simulink model "SOE_H2_DRI_plant"  (R2023b)
settings: Solver=ode15s  StartTime=0.0  StopTime=3600*24*8759
values from neighbouring files (symbols this model uses):
  a_b = 6*(1-eps_bed)/(r_p*2)    (= 200)    [H2_DRI_plant_loader.m]
  A_furnace = pi*r_furnace^2    (= 23.7582944428)    [H2_DRI_plant_loader.m]
  A_furnace_pel = A_furnace*(1-eps_bed)    (= 11.8791472214)    [H2_DRI_plant_loader.m]
  A_wall = (2*pi*r_furnace*dz)    (= 1.1674837564)    [H2_DRI_plant_loader.m]
  c_CH4init = interp1([1:1:length(c_CH4init)],c_CH4init, linspace(1,length(c_CH4init),n_furnace))    [H2_DRI_plant_loader.m]    (also in inital_conditions.m = out.CH4_conc.data(end,:); initcond_H2.mat = [9.94099064213e-45 -4.26076213273e-25 -4.27813906239e-25 -4.; initcond_H2_PEM.mat = [4.30667282687e-45 4.29087427587e-45 3.8700760922e-45 3.7994)
  c_Cinit = interp1([1:1:length(c_Cinit)],c_Cinit, linspace(1,length(c_Cinit),n_furnace))    [H2_DRI_plant_loader.m]    (also in inital_conditions.m = out.C_conc.data(end,:); initcond_H2.mat = [1.45956980986e-305 6.99081092012e-307 8.03725154841e-309 -3; initcond_H2_PEM.mat = [1.92191536232e-321 1.91203404941e-321 1.97132192691e-321 1.)
  c_CO2init = interp1([1:1:length(c_CO2init)],c_CO2init, linspace(1,length(c_CO2init),n_furnace))    [H2_DRI_plant_loader.m]    (also in inital_conditions.m = out.CO2_conc.data(end,:); initcond_H2.mat = [1.40671287015e-53 9.99429922421e-25 1.00349747704e-24 1.007; initcond_H2_PEM.mat = [4.30579616214e-45 4.28998535938e-45 3.86916279543e-45 3.798)
  c_COinit = interp1([1:1:length(c_COinit)],c_COinit, linspace(1,length(c_COinit),n_furnace))    [H2_DRI_plant_loader.m]    (also in inital_conditions.m = out.CO_conc.data(end,:); initcond_H2.mat = [8.62168160047e-54 2.62488347241e-25 2.63562031881e-25 2.646; initcond_H2_PEM.mat = [-1.41770643933e-43 -1.41248114323e-43 -1.27321677334e-43 -1)
  c_Fe2O3init = interp1([1:1:length(c_Fe2O3init)],c_Fe2O3init, linspace(1,length(c_Fe2O3init),n_furnace))    [H2_DRI_plant_loader.m]    (also in inital_conditions.m = out.Fe2O3_conc.data(end,:); initcond_H2.mat = [-0.0576294325141 -0.0562977053664 -0.0549879883395 -0.05369; initcond_H2_PEM.mat = [-0.0421766495112 -0.0410731169681 -0.0399918101679 -0.03893)
  c_Fe3O4init = interp1([1:1:length(c_Fe3O4init)],c_Fe3O4init, linspace(1,length(c_Fe3O4init),n_furnace))    [H2_DRI_plant_loader.m]    (also in inital_conditions.m = out.Fe3O4_conc.data(end,:); initcond_H2.mat = [0.0460784397936 0.0452182842983 0.0443654100081 0.043519007; initcond_H2_PEM.mat = [0.0345314201173 0.0338401633931 0.0331554273597 0.032476466)
  c_Feinit = interp1([1:1:length(c_Feinit)],c_Feinit, linspace(1,length(c_Feinit),n_furnace))    [H2_DRI_plant_loader.m]    (also in inital_conditions.m = out.Fe_conc.data(end,:); initcond_H2.mat = [2291.15615825 2257.57098555 2219.35021937 2176.85237423 213; initcond_H2_PEM.mat = [2291.15370188 2257.40533074 2219.07663621 2176.56351656 213)
  c_FeOinit = interp1([1:1:length(c_FeOinit)],c_FeOinit, linspace(1,length(c_FeOinit),n_furnace))    [H2_DRI_plant_loader.m]    (also in inital_conditions.m = out.FeO_conc.data(end,:); initcond_H2.mat = [120.587032003 163.793602795 212.96382844 267.636483226 327.; initcond_H2_PEM.mat = [120.587036941 164.003608886 213.312732219 268.005087273 327)
  c_H2init = interp1([1:1:length(c_H2init)],c_H2init, linspace(1,length(c_H2init),n_furnace))    [H2_DRI_plant_loader.m]    (also in inital_conditions.m = out.H2_conc.data(end,:); initcond_H2.mat = [22.889073739 22.8842667021 22.8746324515 22.8599710419 22.8; initcond_H2_PEM.mat = [17.1469199078 17.1645959742 17.1787956185 17.1891948084 17.)
  c_H2Oinit = interp1([1:1:length(c_H2Oinit)],c_H2Oinit, linspace(1,length(c_H2Oinit),n_furnace))    [H2_DRI_plant_loader.m]    (also in inital_conditions.m = out.H2O_conc.data(end,:); initcond_H2.mat = [2.19324064628 2.2939246227 2.40633645516 2.52967076126 2.66; initcond_H2_PEM.mat = [0.652099757837 0.728496202531 0.813916572535 0.907739128718)
  c_N2init = interp1([1:1:length(c_N2init)],c_N2init, linspace(1,length(c_N2init),n_furnace))    [H2_DRI_plant_loader.m]    (also in inital_conditions.m = out.N2_conc.data(end,:); initcond_H2.mat = [0.439764167248 0.441445162144 0.443247144888 0.445152489232; initcond_H2_PEM.mat = [0.271051060899 0.272483637209 0.274000693264 0.275587826454)
  cCarbon = 180/1000    (= 0.18)    [H2_DRI_plant_loader.m]
  CCcomp = 6151202*Pcomp^0.71    (= 33253176.5742)    [H2_DRI_plant_loader.m]
  CCeaf = 160*ls_prod_kg*8760/1000    (= 151726003.2)    [H2_DRI_plant_loader.m]
  CCelect = CC_elect*MWelect*1000    (= 480904000)    [H2_DRI_plant_loader.m]
  CCfur = 228860*Qfurnace^0.7848    (= 4163876.6695)    [H2_DRI_plant_loader.m]
  CCpsa = 30622*m_O2^0.6357    (= 6771939.09833)    [H2_DRI_plant_loader.m]
  CCsf = 250*ls_prod_kg*8760/1000    (= 237071880)    [H2_DRI_plant_loader.m]
  cLime = 100/1000    (= 0.1)    [H2_DRI_plant_loader.m]
  cNG = 7    [H2_DRI_plant_loader.m]
  CO2_diff_prop = [MM_CO2, 26.9]    [H2_DRI_plant_loader.m]
  CO_diff_prop = [MM_CO, 18.9]    [H2_DRI_plant_loader.m]
  D_metal = 0.5*I_metal    (= -0.0319284802043)    [H2_DRI_plant_loader.m]
  DRIsteel_conv = 1.075    [H2_DRI_plant_loader.m]
  dz = (h_furnace/(n_furnace-1))    (= 0.0675675675676)    [H2_DRI_plant_loader.m]
  EAF_elec_req = 375    [H2_DRI_plant_loader.m]
  eps_bed = 0.5    [H2_DRI_plant_loader.m]
  eta_comb = 0.8    [H2_DRI_plant_loader.m]
  eta_isen = 0.75    [H2_DRI_plant_loader.m]
  eta_motor = 0.95    [H2_DRI_plant_loader.m]
  H2_diff_prop = [MM_H2, 2.31*2]    [H2_DRI_plant_loader.m]
  H2O_diff_prop = [MM_H2O, 13.1]    [H2_DRI_plant_loader.m]
  H2only = true    [H2_DRI_plant_loader.m]
  hot_standby_eff = 0.009    [H2_DRI_plant_loader.m]
  I_metal = P_metal/tau_metal    (= -0.0638569604087)    [H2_DRI_plant_loader.m]
  Kd = 0.00728    [H2_DRI_plant_loader.m]
  Kmetal = -0.0435    [H2_DRI_plant_loader.m]
  labor_cost = 19*DRI_prod_kg/3600/1000 + 53*ls_prod_kg/3600/1000    (= 2.20779)    [H2_DRI_plant_loader.m]
  m_O2rate = 45.072    [H2_DRI_plant_loader.m]
  MM_C = 12.011/1000    (= 0.012011)    [H2_DRI_plant_loader.m]
  MM_CH4 = 16.04    [H2_DRI_plant_loader.m]
  MM_CO = 28.01    [H2_DRI_plant_loader.m]
  MM_CO2 = 44.01    [H2_DRI_plant_loader.m]
  MM_Fe = 55.845/1000    (= 0.055845)    [H2_DRI_plant_loader.m]    (also in iron_props.m)
  MM_Fe2O3 = 159.69/1000    (= 0.15969)    [H2_DRI_plant_loader.m]    (also in iron_props.m)
  MM_Fe3O4 = 231.53/1000    (= 0.23153)    [H2_DRI_plant_loader.m]    (also in iron_props.m = 0.25153)
  MM_FeO = 71.844/1000    (= 0.071844)    [H2_DRI_plant_loader.m]    (also in iron_props.m)
  MM_H2 = 2.016    [H2_DRI_plant_loader.m]
  MM_H2O = 18.015    [H2_DRI_plant_loader.m]
  MM_N2 = 28.013    [H2_DRI_plant_loader.m]
  MWelect = 240.452    [H2_DRI_plant_loader.m]
  MWhNGeaf = 0.08792    [H2_DRI_plant_loader.m]
  n_furnace = 75    [H2_DRI_plant_loader.m]
  ndot_H2O_feed = linspace(35, 155, n_loops)    [RTO_model_datapoints.m]
  ndot_path = ndot_path(:,3)    [H2_DRI_plant_loader.m]
  ndotin = 2706    [H2_DRI_plant_loader.m]
  nr1init = interp1([1:1:length(nr1init)],nr1init, linspace(1,length(nr1init),n_furnace))    [H2_DRI_plant_loader.m]    (also in inital_conditions.m = out.nr1.data(end,:); initcond_H2.mat = [17138.9259823 17138.9192887 17138.9127057 17138.9062259 171; initcond_H2_PEM.mat = [17138.8483125 17138.8427658 17138.8373309 17138.8319998 171)
  nr2init = interp1([1:1:length(nr2init)],nr2init, linspace(1,length(nr2init),n_furnace))    [H2_DRI_plant_loader.m]    (also in inital_conditions.m = out.nr2.data(end,:); initcond_H2.mat = [11425.7909148 11425.7894343 11425.7880023 11425.7866166 114; initcond_H2_PEM.mat = [11425.7791649 11425.7778635 11425.776614 11425.7754137 1142)
  nr3init = interp1([1:1:length(nr3init)],nr3init, linspace(1,length(nr3init),n_furnace))    [H2_DRI_plant_loader.m]    (also in inital_conditions.m = out.nr3.data(end,:); initcond_H2.mat = [32930.1678524 32447.4572478 31898.1205118 31287.3104766 306; initcond_H2_PEM.mat = [32930.1325476 32445.0763361 31894.188375 31283.1588034 3061)
  oxy_eff_tonne = 0.803    [H2_DRI_plant_loader.m]
  P_g_sp = 101325*2.5    (= 253312.5)    [H2_DRI_plant_loader.m]
  P_metal = tau_metal/(Kmetal*tau_metal_desired)    (= -735.632183908)    [H2_DRI_plant_loader.m]
  pandcdata = csvread('caiso_lmp_carbon_clean.csv', 1, 1)    [H2_DRI_plant_loader.m]
  R = 8.314    [Bou.m]    (also in H2_DRI_plant_loader.m; MD.m; SMR.m; USCM_CO.m)
  r_furnace = 2.75    [H2_DRI_plant_loader.m]
  r_p = 15e-3/2    (= 0.0075)    [H2_DRI_plant_loader.m]
  rho_p = 3528    [H2_DRI_plant_loader.m]
  SOEeff = 37.5    [H2_DRI_plant_loader.m]
  stack_replace = 3.25    [H2_DRI_plant_loader.m]
  T_gin = 950 + 273    (= 1223)    [H2_DRI_plant_loader.m]
  T_ginit = interp1([1:1:length(T_ginit)],T_ginit, linspace(1,length(T_ginit),n_furnace))    [H2_DRI_plant_loader.m]    (also in inital_conditions.m = out.T_g.data(end,2:end); initcond_H2.mat = [1193.47241077 1188.60147936 1183.4413554 1178.04610025 1172; initcond_H2_PEM.mat = [1213.62674902 1206.86882145 1199.80656651 1192.51337179 118)
  T_sin = 10 + 273    (= 283)    [H2_DRI_plant_loader.m]
  T_sinit = interp1([1:1:length(T_sinit)],T_sinit, linspace(1,length(T_sinit),n_furnace))    [H2_DRI_plant_loader.m]    (also in inital_conditions.m = out.T_s.data(end,1:end-1); initcond_H2.mat = [1188.32225462 1183.11411515 1177.66723955 1172.0331792 1166; initcond_H2_PEM.mat = [1207.76768382 1200.67884676 1193.34151616 1185.82650883 117)
  tau = 1    [H2_DRI_plant_loader.m]
  tau_d = 3600    [H2_DRI_plant_loader.m]
  tau_metal = 3.2*3600    (= 11520)    [H2_DRI_plant_loader.m]
  taxes = tax_rate*TIC/8760/3600    [H2_DRI_plant_loader.m]
  V_g = (4/3)*pi*r_p^3*n_pellets_dz*(eps_bed/(1-eps_bed))    (= 0.802645082526)    [H2_DRI_plant_loader.m]
  V_p = 4/3*pi*r_p^3    (= 1.76714586764e-06)    [H2_DRI_plant_loader.m]
  V_s = (4/3)*pi*r_p^3*n_pellets_dz    (= 0.802645082526)    [H2_DRI_plant_loader.m]
  w_Cin = 0    [H2_DRI_plant_loader.m]
  w_Fe2O3in = 0.9665    [H2_DRI_plant_loader.m]
  w_Fe3O4in = 0    [H2_DRI_plant_loader.m]
  w_Fein = 0    [H2_DRI_plant_loader.m]
  w_FeOin = 0    [H2_DRI_plant_loader.m]
  w_Ganin = 0.0335    [H2_DRI_plant_loader.m]
  x_H2in = 0.90    (= 0.9)    [H2_DRI_plant_loader.m]
  x_H2Oin = 0.085    [H2_DRI_plant_loader.m]
  x_N2in = 0.015    [H2_DRI_plant_loader.m]
undefined symbols (not defined in the file or in its folder): CCbop
libraries: slpidlib x2
(part 3 of 3)

== matlab function SOE_H2_DRI_plant/DRI Shaft Furnace/solid_conc ==
  data: rho_Fe2O3in output; w_Fe2O3 input; w_Fe3O4 input; w_FeO input; w_Fe input; w_C input; w_Gan input; m_solid input; rho_Fe3O4in output; rho_FeOin output; A_furnace parameter; rho_Fein output; rho_Cin output; rho_Ganin output; u_sin output; rho_p parameter; eps_bed parameter; pellet_flow output; r_p parameter
function [rho_Fe2O3in, rho_Fe3O4in, rho_FeOin, rho_Fein, rho_Cin, rho_Ganin, u_sin, pellet_flow] = solid_conc(w_Fe2O3, w_Fe3O4, w_FeO, w_Fe, w_C, w_Gan, m_solid, A_furnace,rho_p, eps_bed, r_p)

%toal mass concentration using ped porosity and density of pellet
rho_bedin = rho_p; %kg/^3 of SOLID

%mass concentrations of each iron species in
rho_Fe2O3in = rho_bedin * w_Fe2O3; %kg/m^3 of pellet
rho_Fe3O4in = rho_bedin * w_Fe3O4; %kg/m^3 of pellet
rho_FeOin = rho_bedin * w_FeO; %kg/m^3 of pellet
rho_Fein = rho_bedin * w_Fe; %kg/m^3 of pellet
rho_Cin = rho_bedin * w_C; %kg/m^3 of pellet
rho_Ganin = rho_bedin * w_Gan; %kg/m^3 of pellet


%vol_flow = m_solid/(rho_bedin*(1-eps_bed)); %m^3 total/s

u_sup = m_solid/(rho_p*A_furnace);%*(1-eps_bed));

            
u_sin = u_sup/(1-eps_bed);

%interstitial velocity of mass flow, m/s
%u_sin = m_solid/rho_bedin/(A_furnace*(1-eps_bed));


%check this!
pellet_flow = (3*m_solid)/(4*pi*r_p^3*rho_bedin); %pellets/s

== matlab function SOE_H2_DRI_plant/Electrolyzer/SOE ==
  data: T_gin input; ndot_in input; x_H2in input; x_H2Oin input; x_N2in input; T_gout output; SOEeff parameter; ndot_out output; x_H2out output; x_H2Oout output; x_N2out output; ndot_O2_prod output; MM_H2 parameter; MM_H2O parameter; MM_N2 parameter; MWelect output
function [T_gout, ndot_out, x_H2out, x_H2Oout, x_N2out, ndot_O2_prod, MWelect] = SOE(T_gin, ndot_in, x_H2in, x_H2Oin, x_N2in, SOEeff, MM_H2, MM_H2O, MM_N2)

% mdot_H2_prod = MWelect/(SOEeff*3.6); % kg/s H2 prod
% ndot_H2_prod = mdot_H2_prod/(MM_H2/1000); %mol/s H2 prod
% 
% ndot_O2_prod = 0.5*ndot_H2_prod; %mol/s H2 prod
% ndot_H2O_react = ndot_H2_prod;
% 
% 
% moles_H2 = ndot_in*x_H2in + ndot_H2_prod;
% moles_H2O = ndot_in*x_H2Oin - ndot_H2O_react;
% moles_N2 = ndot_in*x_N2in ;

ndot_out = ndot_in;
x_H2out = 0.89;

ndot_H2_prod = ndot_out*x_H2out - ndot_in*x_H2in;

ndot_O2_prod = 0.5*ndot_H2_prod; %mol/s H2 prod
ndot_H2O_react = ndot_H2_prod;

moles_H2O = ndot_in*x_H2Oin - ndot_H2O_react;
moles_N2 = ndot_in*x_N2in ;


x_H2Oout = moles_H2O/ndot_out;
x_N2out = moles_N2/ndot_out;

T_gout = T_gin + 15;

% mdot_H2_prod = MWelect/(SOEeff*3.6); % kg/s H2 prod
mdot_H2_prod = ndot_H2_prod*MM_H2/1000; %kg/s H2 produced

MWelect = mdot_H2_prod*(SOEeff*3.6); %MW required to react this much

== matlab function SOE_H2_DRI_plant/Splitter/splitter ==
  data: ndotin input; purgefraction input; ndot_comp output; ndot_purge output
function [ndot_comp, ndot_purge] = splitter(ndotin, purgefraction)

ndot_purge = purgefraction*ndotin;
ndot_comp = ndotin*(1-purgefraction);

== matlab function SOE_H2_DRI_plant/Recycle Compressor/compressor ==
  data: P_g_sp input; P_gin input; P_gout output; T_gin input; T_gout output; ndot input; x_H2 input; x_H2O input; x_N2 input; MWcomp output; eta_isen parameter; R parameter; eta_motor parameter; MM_H2O parameter; MM_H2 parameter; MM_N2 parameter
function [P_gout, T_gout, MWcomp] = compressor(P_g_sp, P_gin, T_gin, ndot, x_H2, x_H2O, x_N2, eta_isen, R, eta_motor, MM_H2O, MM_H2, MM_N2)

npoly = 1.4;
P_gout = P_g_sp;


mdot = ndot*(x_H2*MM_H2  + x_H2O*MM_H2O + x_N2*MM_N2)/1000; %kg/s
R_g = R/(x_H2*MM_H2  + x_H2O*MM_H2O + x_N2*MM_N2)*1000; %J/kg-K


%%


W = mdot*(npoly/(npoly-1))*R_g*T_gin*((P_gout/P_gin)^((npoly-1)/npoly) - 1);
MWcomp = W/(eta_isen*eta_motor)/1e6;


T_gout = T_gin*(P_gout/P_gin)^((npoly-1)/npoly);

== matlab function SOE_H2_DRI_plant/Direct Injection Steam Generator/MATLAB Function ==
  data: P_f input; P_gout output; T_gout output; T_f input; ndot_f input; ndotout output; x_H2out output; x_H2Oout output; x_N2out output; P_r input; T_r input; ndot_r input; x_H2_r input; x_H2O_r input; x_N2_r input; MM_H2 parameter; MM_N2 parameter; MM_H2O parameter
function [P_gout, T_gout, ndotout, x_H2out, x_H2Oout, x_N2out] ...
    = steam_gen(P_f, T_f, ndot_f,...
               P_r, T_r, ndot_r, x_H2_r, x_H2O_r, x_N2_r, MM_H2, MM_N2, MM_H2O)

ndotout = ndot_f + ndot_r;

%T_gout = T_r; %need to update using specific heats

P_gout = (ndot_f*P_f + ndot_r*P_r)/(ndotout);

moles_H2 = ndot_r*x_H2_r;
moles_H2O = ndot_r*x_H2O_r + ndot_f;
moles_N2 = ndot_r*x_N2_r ;

x_H2out = moles_H2/ndotout;
x_H2Oout = moles_H2O/ndotout;
x_N2out = moles_N2/ndotout;

%% Recycle Stream

mdot_r = ndot_r*(x_H2_r*MM_H2 + x_N2_r*MM_N2 + x_H2O_r*MM_H2O)/1000; %kg/s

% Weight fractions of each gas species
w_tot_r = (x_H2_r*MM_H2 + x_H2O_r*MM_H2O + x_N2_r*MM_N2);

w_H2_r = x_H2_r*MM_H2/w_tot_r;
w_H2O_r = x_H2O_r*MM_H2O /w_tot_r;
w_N2_r = x_N2_r*MM_N2/w_tot_r;

w_fracs_r = [w_H2_r, w_H2O_r, w_N2_r]; % Create a vector of weight fractions for the prop_mix function

% Get properties from CoolProp interpolation based on temp of gas in
[H_H2, mu_H2, k_H2, C_H2] = hydrogen(T_r);
[H_H2O, mu_H2O, k_H2O, C_H2O] = water(T_r);
[H_N2, mu_N2, k_N2, C_N2] = nitrogen(T_r);


% Create vectors of properties for prop_mix function
Hs = [H_H2, H_H2O, H_N2];
mus = [mu_H2, mu_H2O, mu_N2];
ks = [k_H2, k_H2O, k_N2];
Cps = [C_H2, C_H2O, C_N2];

% get vicosicty and specific heat of gas mixture in
[H_r, ~, ~,  ~] = prop_mix(Hs, mus, ks, Cps, w_fracs_r);

h_r = H_r*mdot_r; % W, enthalpy of recycle stream

%% Water Stream

[H_f, ~, ~,~] = water(T_f);
mdot_f = ndot_f*MM_H2O/1000;
h_f = H_f*mdot_f; % W, enthalpy of feed stream

%% Mixed Enthalpy

H_mix_target = (h_r + h_f)/(mdot_r + mdot_f); %J/kg

%% Out Enthalpy

mdotout = ndotout*(x_H2out*MM_H2 + x_N2out*MM_N2 + x_H2Oout*MM_H2O)/1000; %kg/s

% Weight fractions of each gas species
w_totout = (x_H2out*MM_H2 + x_H2Oout*MM_H2O + x_N2out*MM_N2);

w_H2out = x_H2out*MM_H2/w_totout;
w_H2Oout = x_H2Oout*MM_H2O /w_totout;
w_N2out = x_N2out*MM_N2/w_totout;

w_fracsout = [w_H2out, w_H2Oout, w_N2out]; % Create a vector of weight fractions for the prop_mix function

T_low = 100+273;
T_high = 1000;
tol = 1; 
max_iter = 10000;

T_gout = bisection_method(T_low, T_high, tol, max_iter, w_fracsout, H_mix_target);

== matlab function SOE_H2_DRI_plant/DRI Shaft Furnace/Mixer/MATLAB Function ==
  data: P_gin_f input; P_gout output; T_gout output; T_gin_f input; ndotin_f input; x_H2in_f input; x_H2Oin_f input; x_N2in_f input; x_COin_f input; x_CO2in_f input; x_CH4in_f input; ndotout output; x_H2out output; x_H2Oout output; x_N2out output; x_COout output; x_CO2out output; x_CH4out output; ndotin_N2extra input
function [P_gout, T_gout, ndotout, x_H2out, x_H2Oout, x_N2out, x_COout, x_CO2out, x_CH4out] ...
    = mixer(P_gin_f, T_gin_f, ndotin_f, x_H2in_f, x_H2Oin_f, x_N2in_f, x_COin_f, x_CO2in_f, x_CH4in_f, ndotin_N2extra)

ndotout = ndotin_f + ndotin_N2extra;

T_gout = T_gin_f; %need to update using specific heats

P_gout = P_gin_f;

moles_H2 = ndotin_f*x_H2in_f;
moles_H2O = ndotin_f*x_H2Oin_f;
moles_N2 = ndotin_f*x_N2in_f + ndotin_N2extra;
moles_CO = ndotin_f*x_COin_f;
moles_CO2 = ndotin_f*x_CO2in_f;
moles_CH4 = ndotin_f*x_CH4in_f;

x_H2out = moles_H2/ndotout;
x_H2Oout = moles_H2O/ndotout;
x_N2out = moles_N2/ndotout;
x_COout = moles_CO/ndotout;
x_CO2out = moles_CO2/ndotout;
x_CH4out = moles_CH4/ndotout;

== matlab function SOE_H2_DRI_plant/Combustion Furnace/MATLAB Function ==
  data: ndot input; x_H2 input; x_H2O input; x_N2 input; T_g input; Q_heat output; T_gsp input; MM_H2O parameter; MM_H2 parameter; MM_N2 parameter; mdot output; Cp_g output
function [Q_heat, mdot, Cp_g] = furnace(ndot, x_H2, x_H2O, x_N2, T_g, T_gsp, MM_H2O, MM_H2, MM_N2)

T_g_mid = (T_g + T_gsp)/2;

mdot = ndot*(x_H2*MM_H2 + x_H2O*MM_H2O+ x_N2*MM_N2)/1000; %kg/s

% Weight fractions of each gas species
w_totin = (x_H2*MM_H2 + x_H2O*MM_H2O + x_N2*MM_N2);

w_H2in = x_H2*MM_H2/w_totin;
w_H2Oin = x_H2O*MM_H2O /w_totin;
w_N2in = x_N2*MM_N2/w_totin;


w_fracs = [w_H2in, w_H2Oin, w_N2in]; % Create a vector of weight fractions for the prop_mix function

% Get properties from CoolProp interpolation based on temp of gas in
[rho_H2, mu_H2, k_H2, C_H2] = hydrogen(T_g_mid);
[rho_H2O, mu_H2O, k_H2O, C_H2O] = water(T_g_mid);
[rho_N2, mu_N2, k_N2, C_N2] = nitrogen(T_g_mid);


% Create vectors of properties for prop_mix function
rhos = [rho_H2, rho_H2O, rho_N2];
mus = [mu_H2, mu_H2O, mu_N2];
ks = [k_H2, k_H2O, k_N2];
Cps = [C_H2, C_H2O, C_N2];

% get vicosicty and specific heat of gas mixture in
[~, ~, ~,  Cp_g] = prop_mix(rhos, mus, ks, Cps, w_fracs);

Q_heat = mdot*Cp_g*(T_gsp - T_g)/1e6;

== matlab function SOE_H2_DRI_plant/Combustion Furnace/MATLAB Function1 ==
  data: ndot_p input; Q_purge output; x_H2_p input; x_H2O_p input; x_N2_p input; MM_H2O parameter; MM_H2 parameter; MM_N2 parameter; mdot_p output
function [Q_purge, mdot_p] = purge_comb(ndot_p, x_H2_p, x_H2O_p, x_N2_p, MM_H2O, MM_H2, MM_N2)

Q_purge =  ndot_p*x_H2_p*238440/1e6;

mdot_p = ndot_p*(x_H2_p*MM_H2 + x_H2O_p*MM_H2O+ x_N2_p*MM_N2)/1000; %kg/s

== matlab function SOE_H2_DRI_plant/MATLAB Function ==
  data: LCOE input; elec_CO2rate input; cIO input; pLS input; MWelect input; MWeaf input; MWcomp input; MWpsa input; MWcooltow input; LCOS output; MWng input; MWng_eaf input; m_IO input; m_steel input; carbon_consume input; lime_consume input; CCeaf parameter; CCelect parameter; CCsf parameter; LCOS_bd output; SCE output; SCE_bd output; CCbop parameter; taxes parameter; labor_cost parameter; cNG parameter; cCarbon parameter; cLime parameter; stack_replace parameter; profit output; emissions_profit output; CCfur parameter; CCpsa parameter; CCcomp parameter; cost output; emissions output; MWe output; CCcooltow input
function [LCOS, LCOS_bd, SCE, SCE_bd, profit, emissions_profit, cost, emissions, MWe] = LCOS( LCOE, elec_CO2rate, cIO, pLS, MWelect, MWeaf, MWcomp, MWpsa, MWcooltow, MWng, MWng_eaf,m_IO, m_steel, carbon_consume, lime_consume, ...
    CCeaf, CCelect, CCsf, CCbop, taxes, labor_cost, cNG, cCarbon, cLime, stack_replace, CCfur, CCpsa, CCcomp, CCcooltow)


% m_steel = tonne liquid steel per second

%==========================Variable O&M==============================


io_cost = m_IO*cIO/1000; % $/s, cost of iron ore
MWe = (MWelect+MWeaf+MWcomp+MWpsa+MWcooltow);
elec_cost = (MWelect+MWeaf+MWcomp+MWpsa+MWcooltow)*LCOE/3600; % $/s, cost of electricity
gas_cost = (MWng + MWng_eaf) *3.412*cNG/3600; % $/s, cost of ng

carbon_cost = carbon_consume*cCarbon; %$, cost of carbon
lime_cost = lime_consume*cLime; % cost of lime

stack_cost = MWelect*0.975*stack_replace/3600; % $/s %0.975 is rectifier efficiency - cost to replace stacks


%% LCOS
%CRF = 0.136;
CRF = 0.1019;
%CRF = 0.0776;


CCann = (CCeaf + CCelect + CCsf + CCfur + CCcomp + CCpsa + CCcooltow + CCbop)*CRF;
CC_cost = CCann/(8760*3600); % $/s for plant capital costs

%tax_cost = tax_rate*(CC_cost/CRF +labor_cost); % $/s 

LCOS = (io_cost + elec_cost + gas_cost + CC_cost + taxes + labor_cost + carbon_cost + lime_cost + stack_cost)/m_steel;

cost = (io_cost + elec_cost + gas_cost + CC_cost + taxes + labor_cost + carbon_cost + lime_cost + stack_cost);
revenue = m_steel*pLS;

profit  = revenue - cost;

LCOS_bd = [CCelect*CRF/(8760*3600) CCsf*CRF/(8760*3600) CCeaf*CRF/(8760*3600) ...
    CCfur*CRF/(8760*3600) CCcomp*CRF/(8760*3600) CCpsa*CRF/(8760*3600) CCcooltow*CRF/(8760*3600) CCbop*CRF/(8760*3600)...
    elec_cost  gas_cost  io_cost  carbon_cost + lime_cost + stack_cost labor_cost taxes ]/m_steel;

% ==========================CO2 Emissions==============================
% 
ng_CO2rate = 198; %kg CO2/MWh nat gas -from my 1st paper
ng_CO2rate_us = 47; %kg CO2e nat upstream - from Incentives for Clean Hydrogen Production in the Inflation Reduction Act

lime_CO2rate = 0.05; %kg CO2/kg lime consumed
carbon_CO2rate = 0.98; %kg CO2/kg carbon consumed
io_CO2rate = 0.02; %kg CO2/kg iron ore
pell_CO2rate = 0.16; %kg CO2/kg iron ore
og_CO2rate = 0.101; %kg CO2/kg ls
% 
elec_CO2 = (MWelect+MWeaf+MWcomp+MWpsa+MWcooltow)*elec_CO2rate/3600; %kg CO2/s from electricity
ng_CO2 = (MWng + MWng_eaf)*ng_CO2rate/3600; % kg CO2/s from natural gas combustion
 
EAFog_CO2 = og_CO2rate*m_steel*1000;  %kg CO2/s from combustion of EAF off gas
ng_CO2us = (MWng + MWng_eaf)*ng_CO2rate_us/3600; %kg CO2/s from upstream natural gas use


lime_CO2 = lime_CO2rate*lime_consume; %kg CO2/s from lime production
carbon_CO2 = carbon_CO2rate*carbon_consume; %kg CO2/s from coal/coke production
io_CO2 = io_CO2rate*m_IO; %kg CO2/yr from iron ore mining
pell_CO2 = pell_CO2rate*m_IO;  %kg CO2/yr from iron ore pelletizing
mineralCO2 = lime_CO2 + carbon_CO2 + io_CO2; %kg CO2/yr from mineral production/mining excluding pelletizing

SCE = (elec_CO2 + ng_CO2 + EAFog_CO2 + ng_CO2us + pell_CO2 + mineralCO2)/m_steel/1000; % t CO2e/ t ls
SCE_bd = [ng_CO2  EAFog_CO2  elec_CO2  ng_CO2us   pell_CO2  mineralCO2]/m_steel/1000; % t CO2e/ t ls

emissions = (elec_CO2 + ng_CO2 + EAFog_CO2 + ng_CO2us + pell_CO2 + mineralCO2); %kg/s
emissions_goal = m_steel*1.32*1000; %kg/s

emissions_profit = emissions_goal - emissions;

== matlab function SOE_H2_DRI_plant/Subsystem/EAF ==
  data: m_steel output; m_DRI input; MWeaf output; DRIsteel_conv parameter; EAF_elec_req parameter; MWpsa output; MWng_eaf output; m_O2rate parameter; oxy_eff_tonne parameter; carbon_consume output; lime_consume output; MWhNGeaf parameter
function [m_steel, MWeaf, MWpsa, MWng_eaf, carbon_consume, lime_consume] = eaf(m_DRI, DRIsteel_conv, EAF_elec_req, m_O2rate, oxy_eff_tonne, MWhNGeaf)

m_steel = m_DRI/DRIsteel_conv/1000; %tonne/s steel
m_O2 = m_O2rate*m_steel; %kg/s O2 req
m_O2tonne = m_O2*3.6; % tonne/hr O2 required


MWpsa =  m_O2tonne*oxy_eff_tonne; 

MWeaf = EAF_elec_req*m_steel*3.6; % MWe for EAF

MWng_eaf = MWhNGeaf*m_steel*3600;

%lime and carbon consumption
carbon_consume = 27*m_steel; % kg/s, (kg/tonne ls * tonne_ls)
lime_consume = 50*m_steel; % kg/s, (kg/tonne ls * tonne_ls)

== matlab function SOE_H2_DRI_plant/Direct Injection Steam Generator/MATLAB Function1 ==
  data: time input; ndot_H2O output; ndot_path parameter; t parameter
function ndot_H2O  = interpolator(time, ndot_path, t)

%t = [0:3600:3600*24*31 - 3600]';
ndot_H2O = interp1q(t, ndot_path, time);

== matlab function SOE_H2_DRI_plant/MATLAB Function1 ==
  data: time input; LCOE output; CO2 output; pandcdata parameter; t parameter
function [LCOE, CO2]  = interpolator(time, pandcdata, t)


data = interp1q(t, pandcdata, time);

LCOE = data(1);
CO2 = data(2);
